simulink model "PTB_BatteryElectricVehicle"  (R2018a)
settings: Solver=ode23tb  StartTime=0.0  StopTime=TimeUS06  FixedStep=.001  RelTol=1e-3
model workspace (MAT data in the model file):
  Af = 4
  Cd = 0.3
  DrCycles.C505 = [0 1 2 3 4 5 6 7 8 9 10 11 ... (1012 elements, 506x2)]
  DrCycles.FTP = [0 1 2 3 4 5 6 7 8 9 10 11 ... (4956 elements, 2478x2)]
  DrCycles.UDDS = [0 1 2 3 4 5 6 7 8 9 10 11 ... (2746 elements, 1373x2)]
  DrCycles.HWFET = [0 1 2 3 4 5 6 7 8 9 10 11 ... (1532 elements, 766x2)]
  DrCycles.US06 = [0 1 2 3 4 5 6 7 8 9 10 11 ... (1194 elements, 597x2)]
  DrCycles.US06City = [0 1 2 3 4 5 6 7 8 9 10 11 ... (466 elements, 233x2)]
  DrCycles.US06Hwy = [0 1 2 3 4 5 6 7 8 9 10 11 ... (742 elements, 371x2)]
  I = 1
  Kbr = 5000
  P = 20
  TimeHWFET = 765
  TimeUDDS = 1372
  TimeUS06 = 596
  axle_b = 10
  axle_k = 5000
  bevAxle_wc = 400
  bevNp = 2
  bevNs = 30
  diffRatio = 3.4
  diffRatio1 = 3.4
  motorMaxTorqueNm = [500 500 500 500 500 500 416.666666667 357.142857143 312.5 277.777777778 250 227.272727273 208.333333333 192.307692308 178.571428571 166.666666667]
  motorSpeedRadPs = [0 40 80 120 160 200 240 280 320 360 400 440 480 520 560 600]
  vehicleMass = 1500
  wheelRadius = 0.35
libraries: Wheels_Driver_VehDyn_Lib x3, autolibdatasheetbattery x1, simulink x1, autolibmappedmotor x1, autolibsharedcoupling x1, autolibshareddiff x1
settings Model: PauseTimes=2  Creator=ogden.michael  LastModifiedBy=emarquez
settings DebuggingCC: AlgebraicLoopMsg=none
settings CodeAppCC: StateflowObjectComments=on
settings SimscapeCC: SimscapeNormalizeSystem=off

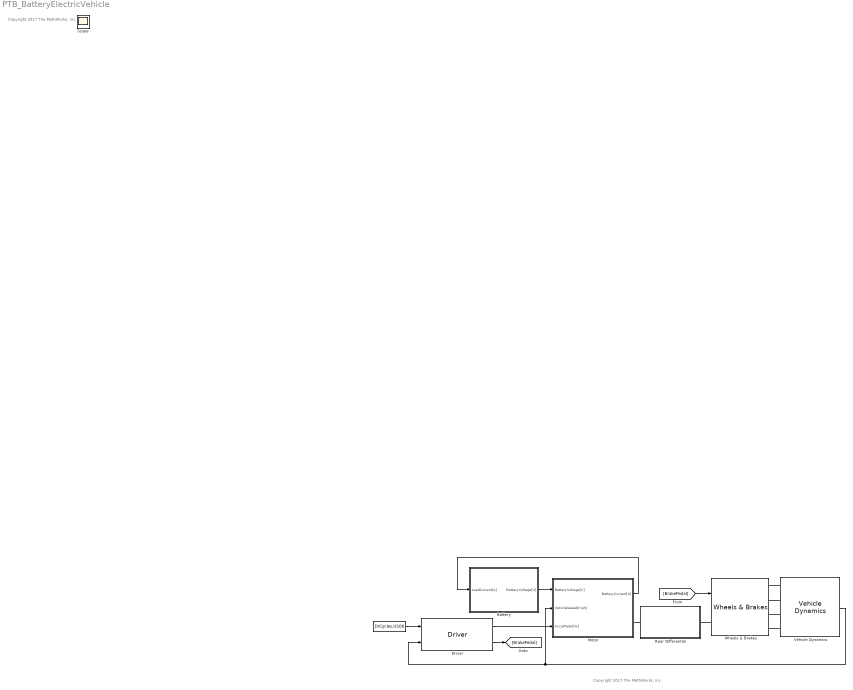
== system PTB_BatteryElectricVehicle ==
  note: Copyright 2017 The MathWorks, Inc.
  note: Copyright 2017 The MathWorks, Inc.
  " " : FromWorkspace  Tag=DriveCycle  VariableName=DrCycles.US06  SampleTime=0
  Battery : Subsystem
  Driver : Wheels_Driver_VehDyn_Lib/Driver
  Motor : Subsystem
  Rear Differential : Subsystem
  Vehicle Dynamics : Wheels_Driver_VehDyn_Lib/Vehicle Dynamics
  Wheels & Brakes : Wheels_Driver_VehDyn_Lib/Wheels & Brakes
  Scope : Scope
  wires:
  " "/1 -> Driver/1
  [BrakePedal] -> Wheels & Brakes/1
  Battery/1(BatteryVoltage[V]) -> Motor/1(BatteryVoltage[V])
  Vehicle Dynamics/1 -> Driver/2, Motor/2(VehicleSpeed[mph])
  Driver/1 -> Motor/3(AccelPedal[%])
  Driver/2 -> [BrakePedal]
  Motor/1(BatteryCurrent[A]) -> Battery/1(LoadCurrent[A])
  connections:
  Motor/RConn1 -- Rear Differential/LConn1
  Wheels & Brakes/LConn1 -- Rear Differential/RConn1
  Vehicle Dynamics/LConn3 -- Wheels & Brakes/RConn3
  Vehicle Dynamics/LConn1 -- Wheels & Brakes/RConn1
  Vehicle Dynamics/LConn4 -- Wheels & Brakes/RConn4
  Vehicle Dynamics/LConn2 -- Wheels & Brakes/RConn2

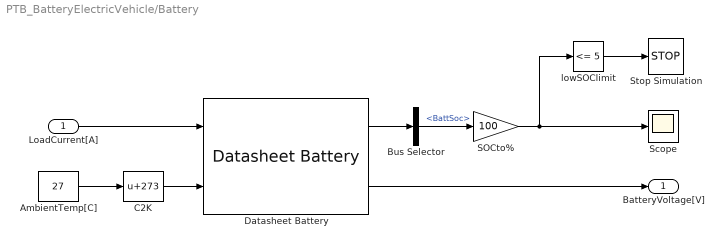
== system PTB_BatteryElectricVehicle/Battery ==
  LoadCurrent[A] : Inport
  AmbientTemp[C] : Constant  Value=27
  Bus Selector : BusSelector  OutputSignals=BattSoc
  C2K : Bias  Bias=273
  Datasheet Battery : autolibdatasheetbattery/Datasheet Battery  CapacityCtrl=Parameter  OutputVlt=Unfiltered  BattChargeMax=100  Em=[2.8 3.228 3.284 3.361 3.408 3.427 3.472 3.477 3.493 3.504 3.516 3.528 3.537 3.545 3.555 3.561 3.566 3.576 3.587 3.589 3.594 3.6 3.608 3.61 3.616 3.619 3.626 3.632 3.637 3.64 3.645 3.646 3.652 3.655 3.658 3.661 3.664 3.668 3.673 3.678 3.68 3.681 3.686 3.692 3.699 3.702 3.705 3.71 3.717 3.723 3.728 3.733 3.735 3.742 3.749 3.755 3.761 3.768 3.773 3.78 3.791 3.798 3.798 3.814 3.818 3.825 3.841 3.846 3.855 3.863 3.877 3.885 3.894 3.907 3.919 3.926 3.935 3.944 3.954 3.964 3.974 3.988 3.998 4.014 4.029 4.034 4.047 4.065 4.074 4.086 4.097 4.131 4.126 4.138 4.15 4.18 4.174 4.187 4.207 4.231 4.221]  CapLUTBp=[0 0.01 0.02 0.03 0.04 0.05 0.06 0.07 0.08 0.09 0.1 0.11 0.12 0.13 0.14 0.15 0.16 0.17 0.18 0.19 0.2 0.21 0.22 0.23 0.24 0.25 0.26 0.27 0.28 0.29 0.3 0.31 0.32 0.33 0.34 0.35 0.36 0.37 0.38 0.39 0.4 0.41 0.42 0.43 0.44 0.45 0.46 0.47 0.48 0.49 0.5 0.51 0.52 0.53 0.54 0.55 0.56 0.57 0.58 0.59 0.6 0.61 0.62 0.63 0.64 0.65 0.66 0.67 0.68 0.69 0.7 0.71 0.72 0.73 0.74 0.75 0.76 0.77 0.78 0.79 0.8 0.81 0.82 0.83 0.84 0.85 0.86 0.87 0.88 0.89 0.9 0.91 0.92 0.93 0.94 0.95 0.96 0.97 0.98 0.99 1]  RInt=[0.008846 0.009319 0.009027 0.00847 0.01032 0.01314;0.006389 0.006554 0.005553 0.005525 0.006043 0.007805;0.004364 0.004101 0.00406 0.003452 0.003846 0.004517;0.002031 0.002563 0.002532 0.00246 0.002716 0.003047;0.001443 0.001825 0.001795 0.001778 0.001924 0.002234;0.0005603 0.0007192 0.0006887 0.0007557 0.0007355 0.001014;0.001028 0.001338 0.001 0.001536 0.001546 0.002789]  BattTempBp=[243.1 253.1 263.1 273.1 283.1 298.1 313.1]  CapSOCBp=[0 0.2 0.4 0.6 0.8 1]  Ns=bevNs  Np=bevNp  BattCapInit=100  Tc=1/1000  Vinit=4.221
      settings: SourceProductName=Powertrain Blockset  SourceProductBaseCode=PW
  SOCto% : Gain  Gain=100
  Scope : Scope
  Stop Simulation : Stop
  lowSOClimit : simulink/Logic and Bit Operations/Compare To Constant  relop=<=  const=5  OutDataTypeStr=boolean
  BatteryVoltage[V] : Outport
  wires:
  Datasheet Battery/1 -> Bus Selector/1
  AmbientTemp[C]/1 -> C2K/1
  Datasheet Battery/2 -> BatteryVoltage[V]/1
  C2K/1 -> Datasheet Battery/2
  SOCto%/1 -> lowSOClimit/1, Scope/1
  Bus Selector/1 -> SOCto%/1  "<BattSoc>"
  LoadCurrent[A]/1 -> Datasheet Battery/1
  lowSOClimit/1 -> Stop Simulation/1

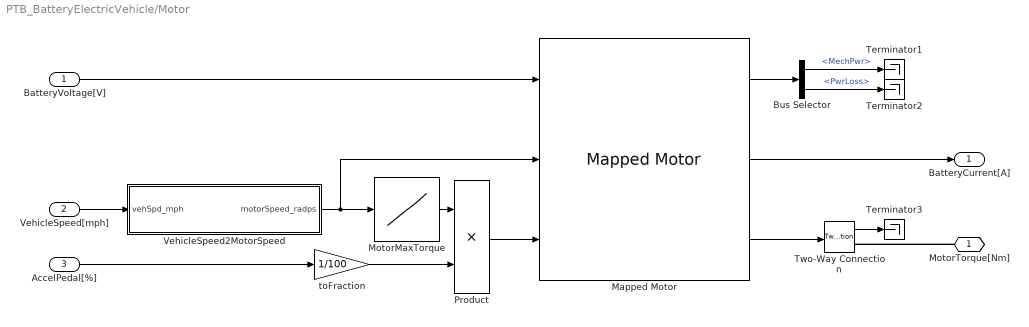
== system PTB_BatteryElectricVehicle/Motor ==
  BatteryVoltage[V] : Inport
  VehicleSpeed[mph] : Inport  Port=2
  AccelPedal[%] : Inport  Port=3
  Bus Selector : BusSelector  OutputSignals=MechPwr,PwrLoss
  Mapped Motor : autolibmappedmotor/Mapped Motor  port_config=Speed  param_by=Tabulated torque-speed envelope  w_t=motorSpeedRadPs  T_t=motorMaxTorqueNm  torque_max=.1  power_max=30  Tc=0.02  param_loss=Single efficiency measurement  eff=100  w_eff=375  T_eff=0.08  Piron=0  Pbase=0  w_eff_bp=[-8000 -4000 0 4000 8000]  T_eff_bp=[0 0.03 0.06 0.09]  losses_table=[1.49 1.67 2.21 3.10; 0.42 0.69 1.14 2.03; 0.06 0.24 0.78 1.68; 0.42 0.69 1.14 2.03; 1.49 1.67 2.21 3.10]  efficiency_table=[95 95 95 95; 95 95 95 95; 95 95 95 95; 95 95 95 95; 95 95 95 95]  J=5e-6  b=1e-5  omega_o=0  T_t_extended=[166.666666666667 178.571428571429 192.307692307692 208.333333333333 227.272727272727 250 277.777777777778 312.5 357.142857142857 416.666666666667 500 500 500 500 500 500 500 500 500 500 500 416.666666666667 357.142857142857 312.5 277.777777777778 250 227.272727272727 208.333333333333 192.307692307692 178.571428571429 166.666666666667]  w_t_extended=[-600 -560 -520 -480 -440 -400 -360 -320 -280 -240 -200 -160 -120 -80 -40 0 40 80 120 160 200 240 280 320 360 400 440 480 520 560 600]  KLossIron=0  KLossCopper=0  x_w_eff_vec=[-8000 -4000 0 4000 8000]  x_T_eff_vec=[-0.09 -0.06 -0.03 0 0.03 0.06 0.09]  x_losses_mat=[3.1 2.21 1.67 1.49 1.67 2.21 3.1;2.03 1.14 0.69 0.42 0.69 1.14 2.03;1.68 0.78 0.24 0.06 0.24 0.78 1.68;2.03 1.14 0.69 0.42 0.69 1.14 2.03;3.1 2.21 1.67 1.49 1.67 2.21 3.1]
      settings: SourceProductName=Powertrain Blockset  SourceProductBaseCode=PW
  MotorMaxTorque : Lookup_n-D  NumberOfTableDimensions=1  BreakpointsForDimension1=motorSpeedRadPs  Table=motorMaxTorqueNm  ExtrapMethod=Clip  InternalRulePriority=Speed  RndMeth=Simplest  InputSameDT=on
  Product : Product
  Terminator1 : Terminator
  Terminator2 : Terminator
  Terminator3 : Terminator
  Two-Way Connectio n : TwoWayConnection
  VehicleSpeed2MotorSpeed : Subsystem
  toFraction : Gain  Gain=1/100
  MotorTorque[Nm] : PMIOPort  Side=Right
  BatteryCurrent[A] : Outport
  wires:
  BatteryVoltage[V]/1 -> Mapped Motor/1
  Mapped Motor/2 -> BatteryCurrent[A]/1
  VehicleSpeed[mph]/1 -> VehicleSpeed2MotorSpeed/1(vehSpd_mph)
  VehicleSpeed2MotorSpeed/1(motorSpeed_radps) -> MotorMaxTorque/1, Mapped Motor/2
  Mapped Motor/1 -> Bus Selector/1
  Two-Way Connectio n/1 -> Terminator3/1
  Product/1 -> Mapped Motor/3
  MotorMaxTorque/1 -> Product/1
  AccelPedal[%]/1 -> toFraction/1
  toFraction/1 -> Product/2
  Bus Selector/2 -> Terminator2/1  "<PwrLoss>"
  Bus Selector/1 -> Terminator1/1  "<MechPwr>"
  Mapped Motor/3 -> Two-Way Connectio n/1
  connections:
  MotorTorque[Nm]/RConn1 -- Two-Way Connectio n/RConn1

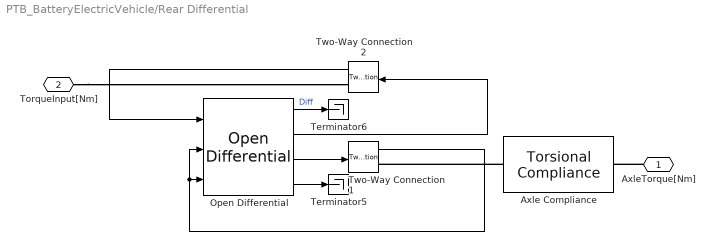
== system PTB_BatteryElectricVehicle/Rear Differential ==
  Axle Compliance : autolibsharedcoupling/Torsional Compliance  port_config=Two-way connection  k=axle_k  b=axle_b  theta_o=0  domega_o=0  omega_c=bevAxle_wc  blkID=0  aMode=1
      settings: SourceProductName=Powertrain Blockset  SourceProductBaseCode=PW
  Open Differential : autolibshareddiff/Open Differential  shaftSwitchMask=To the left of center-line  Ndiff=diffRatio  Jd=.025  bd=1e-3  Jw1=.01  bw1=1e-3  Jw2=.01  bw2=1e-3  omegaw1o=0  omegaw2o=0  maxAbsSpd=5e3
      settings: SourceProductName=Powertrain Blockset  SourceProductBaseCode=PW
  Terminator5 : Terminator
  Terminator6 : Terminator
  Two-Way Connection1 : TwoWayConnection
  Two-Way Connection2 : TwoWayConnection
  AxleTorque[Nm] : PMIOPort  Side=Right
  TorqueInput[Nm] : PMIOPort  Port=2  Side=Left
  wires:
  Open Differential/3 -> Two-Way Connection1/1
  Open Differential/4 -> Terminator5/1
  Open Differential/1 -> Terminator6/1  "Diff"
  Open Differential/2 -> Two-Way Connection2/1
  Two-Way Connection1/1 -> Open Differential/2, Open Differential/3
  Two-Way Connection2/1 -> Open Differential/1
  connections:
  Axle Compliance/LConn1 -- Two-Way Connection1/RConn1
  TorqueInput[Nm]/RConn1 -- Two-Way Connection2/RConn1
  AxleTorque[Nm]/RConn1 -- Axle Compliance/RConn1

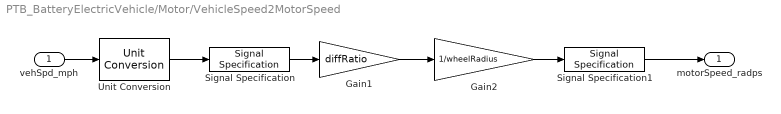
== system PTB_BatteryElectricVehicle/Motor/VehicleSpeed2MotorSpeed ==
  vehSpd_mph : Inport
  Gain1 : Gain  Gain=diffRatio
  Gain2 : Gain  Gain=1/wheelRadius
  Signal Specification : SignalSpecification  Unit=m/s
  Signal Specification1 : SignalSpecification  Unit=rad/s
  Unit Conversion : UnitConversion
  motorSpeed_radps : Outport
  wires:
  Signal Specification1/1 -> motorSpeed_radps/1
  Unit Conversion/1 -> Signal Specification/1
  vehSpd_mph/1 -> Unit Conversion/1
  Signal Specification/1 -> Gain1/1
  Gain1/1 -> Gain2/1
  Gain2/1 -> Signal Specification1/1
